simulink model "Slx003_Jacobians_M1_OptimizeJoint_TTRobot_"  (R2017b)
settings: Solver=FixedStepAuto  StartTime=0  StopTime=20  FixedStep=0.001  RelTol=1e-3
settings Model: Creator=Dell  LastModifiedBy=Dell

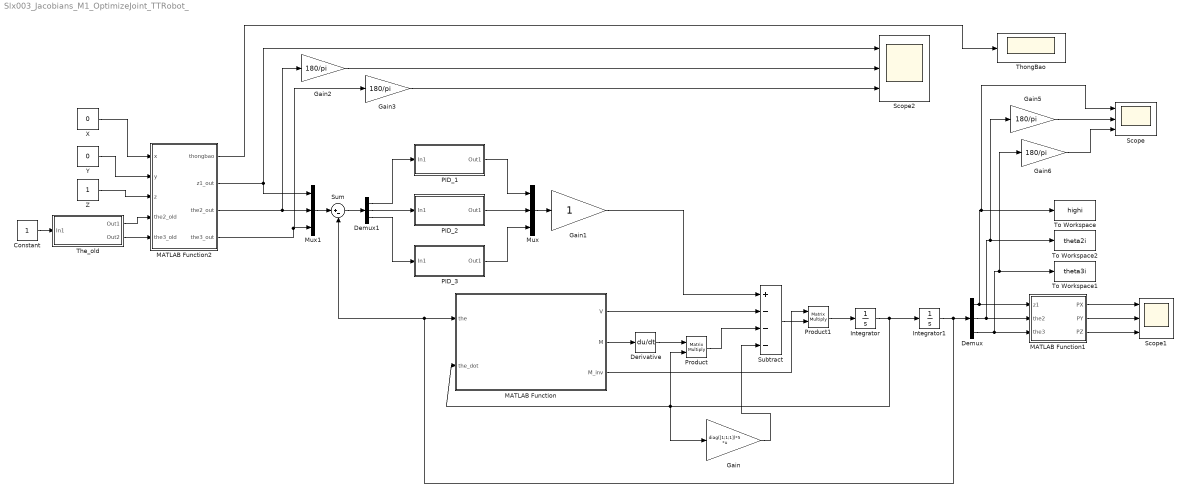
== system Slx003_Jacobians_M1_OptimizeJoint_TTRobot_ ==
  Constant : Constant
  Demux : Demux  Outputs=3
  Demux1 : Demux  Outputs=3
  Derivative : Derivative
  Gain : Gain  Gain=diag([1;1;1])*5  Multiplication=Matrix(K*u)
  Gain1 : Gain
  Gain{2..3,5..6} (4 alike) : Gain  Gain=180/pi
  Integrator : Integrator  InitialCondition=[0; 0; 0]
  Integrator1 : Integrator  InitialCondition=[5; pi/3; pi/4]
  MATLAB Function : MATLAB Function  TreatAsAtomicUnit=on
  MATLAB Function1 : MATLAB Function  TreatAsAtomicUnit=on
  MATLAB Function2 : MATLAB Function  TreatAsAtomicUnit=on
  Mux : Mux  Inputs=3
  Mux1 : Mux  Inputs=3
  PID_1 : Subsystem  mask{Kp=1000, Ki=54, Kd=30}
  PID_2 : Subsystem  mask{Kp=50, Ki=0.1, Kd=1}
  PID_3 : Subsystem  mask{Kp=50, Ki=0.1, Kd=1}
  Product : Product  Multiplication=Matrix(*)
  Product1 : Product  Multiplication=Matrix(*)
  Scope : Scope  NumInputPorts=3
  Scope1 : Scope  NumInputPorts=3
  Scope2 : Scope  NumInputPorts=3
  Subtract : Sum  Inputs=+---
  Sum : Sum  Inputs=|+-
  "The_old " : Subsystem  mask{the2_old=pi/3, the3_old=pi/4}
  ThongBao : Scope
  To Workspace : ToWorkspace  VariableName=highi  SaveFormat=Timeseries  SampleTime=0.1
  To Workspace1 : ToWorkspace  VariableName=theta3i  SaveFormat=Timeseries  SampleTime=0.1
  To Workspace2 : ToWorkspace  VariableName=theta2i  SaveFormat=Timeseries  SampleTime=0.1
  X : Constant  Value=0
  Y : Constant  Value=0
  Z : Constant
  wires:
  MATLAB Function/2(M) -> Derivative/1
  Derivative/1 -> Product/1
  Product/1 -> Subtract/3
  MATLAB Function/1(V) -> Subtract/2
  Subtract/1 -> Product1/2
  MATLAB Function/3(M_inv) -> Product1/1
  Product1/1 -> Integrator/1
  Integrator1/1 -> Sum/2, MATLAB Function/1(the), Demux/1
  Demux/3 -> MATLAB Function1/3(the3), Gain6/1, To Workspace1/1
  Integrator/1 -> Gain/1, Product/2, MATLAB Function/2(the_dot), Integrator1/1
  Gain/1 -> Subtract/4
  Mux/1 -> Gain1/1
  PID_2/1(Out1) -> Mux/2
  PID_3/1(Out1) -> Mux/3
  PID_1/1(Out1) -> Mux/1
  Gain1/1 -> Subtract/1
  Demux1/2 -> PID_2/1(In1)
  Demux1/1 -> PID_1/1(In1)
  Demux1/3 -> PID_3/1(In1)
  Sum/1 -> Demux1/1
  Demux/2 -> MATLAB Function1/2(the2), Gain5/1, To Workspace2/1
  MATLAB Function1/2(PY) -> Scope1/2
  MATLAB Function1/1(PX) -> Scope1/1
  MATLAB Function1/3(PZ) -> Scope1/3
  Mux1/1 -> Sum/1
  Z/1 -> MATLAB Function2/3(z)
  Y/1 -> MATLAB Function2/2(y)
  X/1 -> MATLAB Function2/1(x)
  MATLAB Function2/2(z1_out) -> Scope2/1, Mux1/1
  MATLAB Function2/3(the2_out) -> Gain2/1, Mux1/2
  MATLAB Function2/4(the3_out) -> Gain3/1, Mux1/3
  Gain3/1 -> Scope2/3
  Gain5/1 -> Scope/2
  Demux/1 -> Scope/1, To Workspace/1, MATLAB Function1/1(z1)
  Gain6/1 -> Scope/3
  Gain2/1 -> Scope2/2
  MATLAB Function2/1(thongbao) -> ThongBao/1
  Constant/1 -> "The_old "/1(In1)
  "The_old "/2(Out2) -> MATLAB Function2/5(the3_old)
  "The_old "/1(Out1) -> MATLAB Function2/4(the2_old)

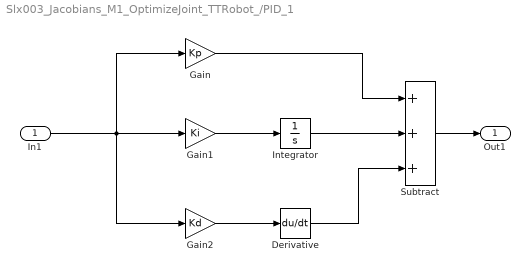
== system Slx003_Jacobians_M1_OptimizeJoint_TTRobot_/PID_1 ==
  In1 : Inport
  Derivative : Derivative
  Gain : Gain  Gain=Kp
  Gain1 : Gain  Gain=Ki
  Gain2 : Gain  Gain=Kd
  Integrator : Integrator
  Subtract : Sum  Inputs=+++
  Out1 : Outport
  wires:
  Gain1/1 -> Integrator/1
  Gain2/1 -> Derivative/1
  Subtract/1 -> Out1/1
  Integrator/1 -> Subtract/2
  Gain/1 -> Subtract/1
  Derivative/1 -> Subtract/3
  In1/1 -> Gain2/1, Gain/1, Gain1/1

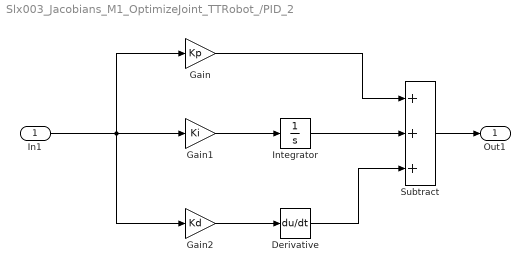
== system Slx003_Jacobians_M1_OptimizeJoint_TTRobot_/PID_2 ==
  In1 : Inport
  Derivative : Derivative
  Gain : Gain  Gain=Kp
  Gain1 : Gain  Gain=Ki
  Gain2 : Gain  Gain=Kd
  Integrator : Integrator
  Subtract : Sum  Inputs=+++
  Out1 : Outport
  wires:
  Gain1/1 -> Integrator/1
  Gain2/1 -> Derivative/1
  Subtract/1 -> Out1/1
  Integrator/1 -> Subtract/2
  Gain/1 -> Subtract/1
  Derivative/1 -> Subtract/3
  In1/1 -> Gain2/1, Gain/1, Gain1/1

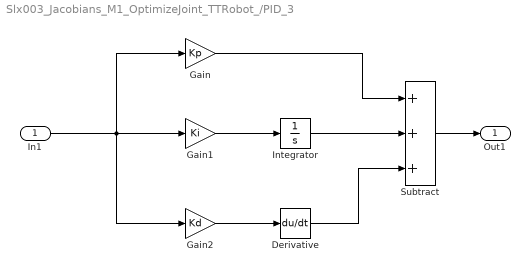
== system Slx003_Jacobians_M1_OptimizeJoint_TTRobot_/PID_3 ==
  In1 : Inport
  Derivative : Derivative
  Gain : Gain  Gain=Kp
  Gain1 : Gain  Gain=Ki
  Gain2 : Gain  Gain=Kd
  Integrator : Integrator
  Subtract : Sum  Inputs=+++
  Out1 : Outport
  wires:
  Gain1/1 -> Integrator/1
  Gain2/1 -> Derivative/1
  Subtract/1 -> Out1/1
  Integrator/1 -> Subtract/2
  Gain/1 -> Subtract/1
  Derivative/1 -> Subtract/3
  In1/1 -> Gain2/1, Gain/1, Gain1/1

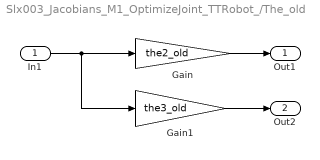
== system Slx003_Jacobians_M1_OptimizeJoint_TTRobot_/The_old  ==
  In1 : Inport
  Gain : Gain  Gain=the2_old
  Gain1 : Gain  Gain=the3_old
  Out1 : Outport
  Out2 : Outport  Port=2
  wires:
  Gain/1 -> Out1/1
  In1/1 -> Gain1/1, Gain/1
  Gain1/1 -> Out2/1

== matlab function Slx003_Jacobians_M1_OptimizeJoint_TTRobot_/MATLAB Function1 ==
  data: z1 input; the2 input; the3 input; PX output; PY output; PZ output
function [PX, PY, PZ] = fcn(z1, the2, the3)
m1=1; m2=1; m3=1; l1=1; l2=1;
c2=cos(the2);
s2=sin(the2);
c3=cos(the3);
s3=sin(the3);
c23=cos(the2 + the3);
s23=sin(the2 + the3);
P_0_EE = [(l2*c23 + l1*c2); (l2*s23 + l1*s2); z1];
PX = P_0_EE(1,1);
PY = P_0_EE(2,1);
PZ = P_0_EE(3,1);

== matlab function Slx003_Jacobians_M1_OptimizeJoint_TTRobot_/MATLAB Function ==
  data: the input; V output; the_dot input; M output; M_inv output
function [V, M, M_inv] = fcn(the, the_dot)
m1=1; m2=1; m3=1; l1=1; l2=1; z1=3;
g0 = [0; 0; -9.81];
%g0 = [0; -9.81; 0];
c2=cos(the(2));
s2=sin(the(2));
c3=cos(the(3));
s3=sin(the(3));
c23=cos(the(2) + the(3));
s23=sin(the(2)+the(3));

P_0_EE = [(l2*c23 + l1*c2); (l2*s23 + l1*s2); z1];
P_0_2 = [l1*c2; l1*s2; z1];
P_0_1 = [0; 0; z1];

J_3 = [0 (-(l2*s23 + l1*s2)) (-l2*s23);...
       0 (l2*c23 + l1*c2)    (l2*c23);...
       1 0                   0];
J_2 = [0 (-l1*s2) 0;...
       0 (l1*c2)  0;...
       1 0        0];
J_1 = [0 0 0;...
       0 0 0;...
       1 0 0];

M = (m1*(J_1')*J_1 + m2*(J_2')*J_2 + m3*(J_3')*J_3) + 0.01*eye(3); %0.01*eye(3) la` he. so' ma sat' truot.
M_inv = inv(M);

dJ1_dz1 = zeros(3,3); %zeros(3,3) la` matrix 3x3 voi' all phan` tu~ la` 0
dJ1_dthe2 = zeros(3,3);
dJ1_dthe3 = zeros(3,3);
dJ2_dz1 = zeros(3,3);
dJ2_dthe2 = [0 -l1*c2 0;...
             0 -l1*s2 0;...
             0 0      0];
dJ2_dthe3 = zeros(3,3); %zeros(3,3) la` matrix 3x3 voi' all phan` tu~ la` 0
dJ3_dz1 = zeros(3,3);
dJ3_dthe2 = [0 (-l2*c23 - l1*c2) -l2*c23;...
             0 (-l2*s23 - l1*s2) -l2*s23;...
             0 0                 0];
dJ3_dthe3 = [0 -l2*c23 -l2*c23;...
             0 -l2*s23 -l2*s23;...
             0 0       0];
         
V1 = (the_dot')*(m1*dJ1_dz1*J_1 + m2*dJ2_dz1*J_2* + m3*dJ3_dz1*J_3)*the_dot;
V2 = (the_dot')*(m1*dJ1_dthe2*J_1 + m2*dJ2_dthe2*J_2* + m3*dJ3_dthe2*J_3)*the_dot;
V3 = (the_dot')*(m1*dJ1_dthe3*J_1 + m2*dJ2_dthe3*J_2* + m3*dJ3_dthe3*J_3)*the_dot;

dP_dthe = (J_2' + J_3')*g0;
V=[V1;V2;V3]-dP_dthe;

== matlab function Slx003_Jacobians_M1_OptimizeJoint_TTRobot_/MATLAB Function2 ==
  data: thongbao output; x input; z1_out output; y input; z input; the2_out output; the3_out output; the2_old input; the3_old input
function [thongbao,z1_out,the2_out,the3_out] = fcn(x, y, z, the2_old, the3_old)
l1=1; l2=1; 
z1_out = z;
the3 = basic_atan2( (2*l1*l2), (0) , (x*x + y*y - l1*l1 - l2*l2));
the3_1 = the3(1,1);
the3_2 = the3(2,1);

the2_1 = basic_atan2( (l2*cos(the3_1) + l1), (l2*sin(the3_1)) , (x));
the2_2 = basic_atan2( (l2*cos(the3_2) + l1), (l2*sin(the3_2)) , (x));
the2_3 = basic_atan2( (l2*sin(the3_1) ), (l2*cos(the3_1) + l1) , (y));
the2_4 = basic_atan2( (l2*sin(the3_2) ), (l2*cos(the3_2) + l1) , (y));

the2 = [the2_1(1,1); the2_1(2,1); the2_2(1,1); the2_2(2,1); the2_3(1,1); the2_3(2,1); the2_4(1,1); the2_4(2,1)];
n=0;
the = [0 0; 0 0];
 for i = 1:2
     for j = 1:4
         PX = l1*cos(the2(j,1)) + l2*cos(the2(j,1)+the3(i,1));
         PY = l1*sin(the2(j,1)) + l2*sin(the2(j,1)+the3(i,1));
         X_tam = abs(PX - x);
         Y_tam = abs(PY - y);
          if((X_tam<=0.0005)&&(Y_tam<=0.0005)&&(n<2))
            n = n+1;
            the(n,1) = (the2(j,1));
            the(n,2) = (the3(i,1));
          end
     end
 end
the2_tam = [the(1,1); the(2,1)];
the3_tam = [the(1,2); the(2,2)];
the2_sosanh = [0;0];
the3_sosanh = [0;0];
the2_tt = [0;0];
the3_tt = [0;0];
total = [0;0];
limit_duong = 110*pi/180;
limit_am = -110*pi/180;
 if( (the2_tam(1,1)>(limit_duong)) || (the2_tam(1,1)<(limit_am)) )
     the2_sosanh(1,1) = 0;
     the2_a = 0;
 else
     the2_sosanh(1,1) = the2_tam(1,1);
     the2_a = 1;
 end
 
 if( (the2_tam(2,1)>(limit_duong)) || (the2_tam(2,1)<(limit_am)) )
     the2_sosanh(2,1) = 0;
     the2_b = 0;
 else
     the2_sosanh(2,1) = the2_tam(2,1);
     the2_b = 1;
 end
 
 if( (the3_tam(1,1)>(limit_duong)) || (the3_tam(1,1)<(limit_am)) )
     the3_sosanh(1,1) = 0;
     the3_a = 0;
 else
     the3_sosanh(1,1) = the3_tam(1,1);
     the3_a = 1;
 end
 
 if( (the3_tam(2,1)>(limit_duong)) || (the3_tam(2,1)<(limit_am)) )
     the3_sosanh(2,1) = 0;
     the3_b = 0;
 else
     the3_sosanh(2,1) = the3_tam(2,1);
     the3_b = 1;
 end
hs_1 = the2_a*the3_a;
hs_2 = the2_b*the3_b;
hs_total = hs_1+hs_2;


 for i = 1:2
     the2_tt(i,1) = abs(the2_sosanh(i,1) - the2_old);
     the3_tt(i,1) = abs(the3_sosanh(i,1) - the3_old);
     total(i,1) = the2_tt(i,1) + the3_tt(i,1);
 end
 
 delta_the = total(1,1) - total(2,1);
 
 if(hs_total == 0)
     the2_out = 0;
     the3_out = 0;
     thongbao = 1;
 else
     thongbao = 0;
     if(((delta_the<=0)&&(hs_1==1))||(hs_2==0))
         the2_out = the(1,1);
         the3_out = the(1,2);
     else
         the2_out = the(2,1);
         the3_out = the(2,2);
     end
 end
